simulink model "DampedOscillator"  (R2017a)
settings: Solver=ode45  StartTime=0.0  StopTime=25  MaxStep=1  RelTol=1e-3  AbsTol=1e-6  EnableMultiTasking=on
PreLoadFcn:
  | b=2;
  | k=3;
  | 
  | assignin('base','D',k);
  | assignin('base','m',5);
  | assignin('base','R',b);
  | assignin('base','x0',0);
  | assignin('base','x0_dot',1);
StopFcn:
  | bh=find_system(gcs,'FindAll','on','BlockType','Scope');
  | for x=1:length(bh)          %close all scope
  |     set_param(bh(x),'Open','off');
  | end
  | for x=1:length(bh)
  |     set_param(bh(x),'Open','on');
  | end
undefined symbols (not defined in the file or in its folder): D, m, R, x0, x0_dot
libraries: simulink x1
settings Model: Creator=aschreib  LastModifiedBy=sdewolsk
settings SolverCC: ZeroCrossControl=EnableAll
settings DataIOCC: LimitDataPoints=on  SaveFormat=Array  SignalLoggingSaveFormat=ModelDataLogs  ReturnWorkspaceOutputs=on
settings OptimizationCC: ExpressionDepthLimit=2147483647  LifeSpan=inf
settings DebuggingCC: UnderspecifiedInitializationDetection=Classic  MergeDetectMultiDrivingBlocksExec=none  SolverPrmCheckMsg=warning  FcnCallInpInsideContextMsg=warning  StateNameClashWarn=warning  SFUnexpectedBacktrackingDiag=warning  SFNoUnconditionalDefaultTransitionDiag=warning  SFExecutionAtInitializationDiag=none
settings HardwareCC: ProdBitPerPointer=32  ProdBitPerSizeT=32  ProdBitPerPtrDiffT=32  ProdLargestAtomicFloat=None  ProdIntDivRoundTo=Undefined  ProdEndianess=Unspecified  ProdWordSize=32  ProdHWDeviceType=32-bit Generic
settings ModelReferenceCC: PropagateSignalLabelsOutOfModel=off
settings GRTTargetCC: TargetLangStandard=C89/C90 (ANSI)  GeneratePreprocessorConditionals=Disable all  CombineOutputUpdateFcns=off  GRTInterface=on
settings ConfigComp: CovMetricSettings=dw  CovHtmlReporting=on  CovSaveCumulativeToWorkspaceVar=on  CovSaveSingleToWorkspaceVar=on  CovExternalEMLEnable=off

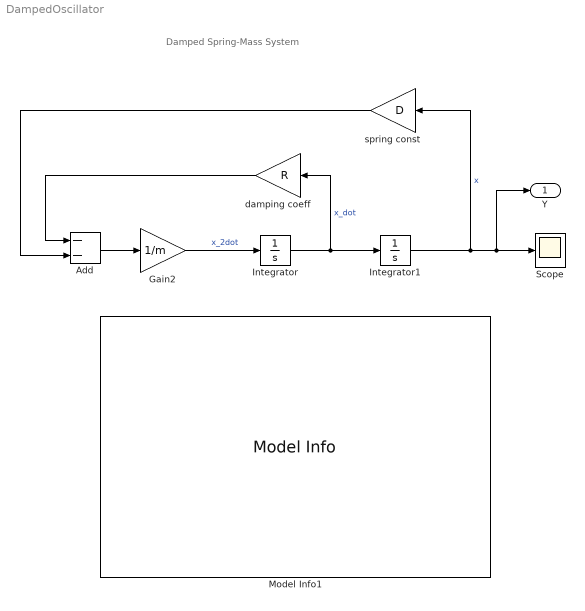
== system DampedOscillator ==
  note: Damped Spring-Mass System
  Add : Sum  Inputs=--
  Gain2 : Gain  Gain=1/m
  Integrator : Integrator  InitialCondition=x0_dot
  Integrator1 : Integrator  InitialCondition=x0
  Model Info1 : simulink/Model-Wide Utilities/Model Info  BlockCM=None  Frame=on  DisplayStringWithTags=|  HorizontalTextAlignment=Left  LeftAlignmentValue=0.02  SourceBlockDiagram=Copy_of_damped_osc_v2  TagMaxNumber=20
      | Ordinary Differential Equation:
      | 
      |   mx'' + Rx' + Dx = 0
      |   => x'' = 1/m (-Rx' - Dx)
      | 
      |   m: mass
      |   R: damping coefficient
      |   D: spring constant
      | 
      | Special cases:
      |   - R = 0: no damping, i.e. harmonic oscillation (yellow)
      |   - D/m > R^2/(4m^2): under damping (purple)
      |   - D/m = R^2/(4m^2): critical damping (turquois)
      |   - D/m < R^2/(4m^2): over damping (red)
  Scope : Scope
  damping coeff : Gain  Gain=R
  spring const : Gain  Gain=D
  Y : Outport
  wires:
  Add/1 -> Gain2/1
  Integrator/1 -> Integrator1/1, damping coeff/1  "x_dot"
  Integrator1/1 -> spring const/1, Y/1, Scope/1  "x"
  damping coeff/1 -> Add/1
  spring const/1 -> Add/2
  Gain2/1 -> Integrator/1  "x_2dot"
